simulink model "Nonterm1"  (Simulink 5.0)
settings: Solver=FixedStepDiscrete  StartTime=0.0  StopTime=10.0  RelTol=1e-3
settings Model: Creator=sofronis  LastModifiedBy=scaife  ExtModeAutoUpdateStatusClock=off  AlgebraicLoopMsg=error

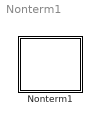
== system Nonterm1 ==
  Nonterm1 : Stateflow chart

== stateflow chart Nonterm1 ==
  state A/
    en: E
  state B
  (default) -> A
  A -> B : E { E }
  events: E local EITHER_EDGE_EVENT
